simulink model "Myp6LinearIntegralObserverFeed"  (R2021b)
settings: Solver=ode4  StartTime=0.0  StopTime=TIME_SIM  FixedStep=STEP_SIZE  RelTol=1e-3
values from neighbouring files (symbols this model uses):
  Aa = [-0.329723564087  0.00108308678514  -14.6666835708; 119.959269051  -1.23669349537  16746.7578957; 1  -0.0103092783505  0]    [LinearModel.mat]
  Bb = [-1.10657474768  0; 0  -0.0018722524695; 0  0]    [LinearModel.mat]
  Bv = [0.0209040137669 0 0]    [LinearModel.mat]
  Dd = [0  0; 0  0.0001229087]    [LinearModel.mat]
  xOP = [1.2671 122.9087 0.00454800621385]    [LinearModel.mat]
undefined symbols (not defined in the file or in its folder): Cc0, Ff, Gg, K_FSF, Ki, L, Ts
settings Model: Creator=tanzc  LastModifiedBy=tanzc
settings DataIOCC: SaveFormat=Array  ReturnWorkspaceOutputs=off

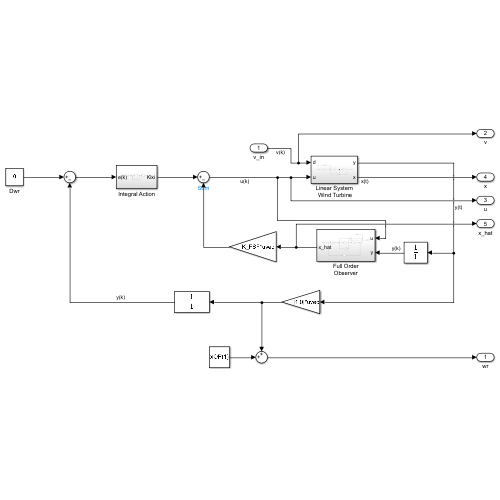
[thumbnail: Simulink's stored preview of the top-level diagram]
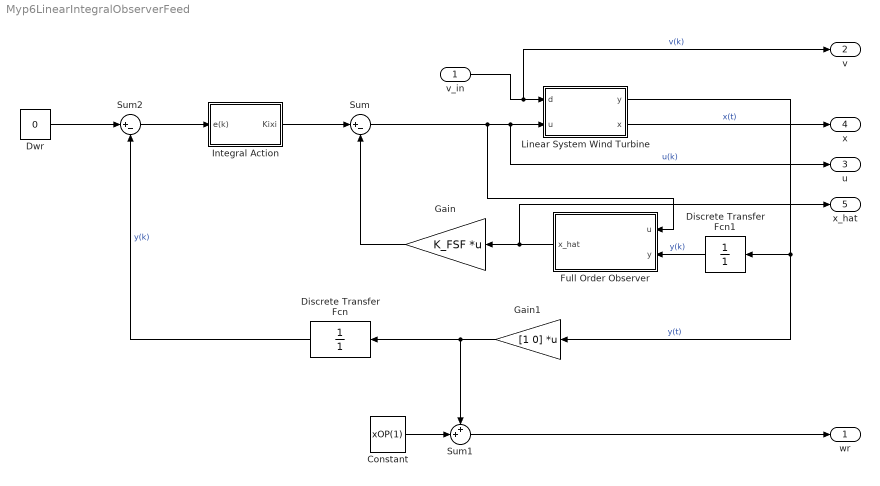
== system Myp6LinearIntegralObserverFeed ==
  v_in : Inport
  Constant : Constant  Value=xOP(1)
  Discrete Transfer Fcn : DiscreteTransferFcn  Denominator=1  SampleTime=Ts
  Discrete Transfer Fcn1 : DiscreteTransferFcn  Denominator=1  SampleTime=Ts
  Dwr : Constant  Value=0  SampleTime=Ts
  Full Order Observer : Subsystem
  Gain : Gain  Gain=K_FSF  Multiplication=Matrix(K*u) (u vector)
  Gain1 : Gain  Gain=[1 0]  Multiplication=Matrix(K*u) (u vector)
  Integral Action : Subsystem
  Linear System Wind Turbine : Subsystem
  Sum : Sum  Inputs=|+-
  Sum1 : Sum  Inputs=++|
  Sum2 : Sum  Inputs=|+-
  wr : Outport
  v : Outport  Port=2
  u : Outport  Port=3
  x : Outport  Port=4
  x_hat : Outport  Port=5
  wires:
  Gain/1 -> Sum/2
  Sum/1 -> Full Order Observer/1(u), Linear System Wind Turbine/2(u), u/1  "u(k)"
  v_in/1 -> v/1, Linear System Wind Turbine/1(d)  "v(k)"
  Dwr/1 -> Sum2/1
  Discrete Transfer Fcn/1 -> Sum2/2  "y(k)"
  Linear System Wind Turbine/1(y) -> Discrete Transfer Fcn1/1, Gain1/1  "y(t)"
  Sum2/1 -> Integral Action/1(e(k))
  Integral Action/1(Kixi) -> Sum/1
  Discrete Transfer Fcn1/1 -> Full Order Observer/2(y)  "y(k)"
  Full Order Observer/1(x_hat) -> x_hat/1, Gain/1
  Gain1/1 -> Sum1/1, Discrete Transfer Fcn/1
  Constant/1 -> Sum1/2
  Sum1/1 -> wr/1
  Linear System Wind Turbine/2(x) -> x/1  "x(t)"

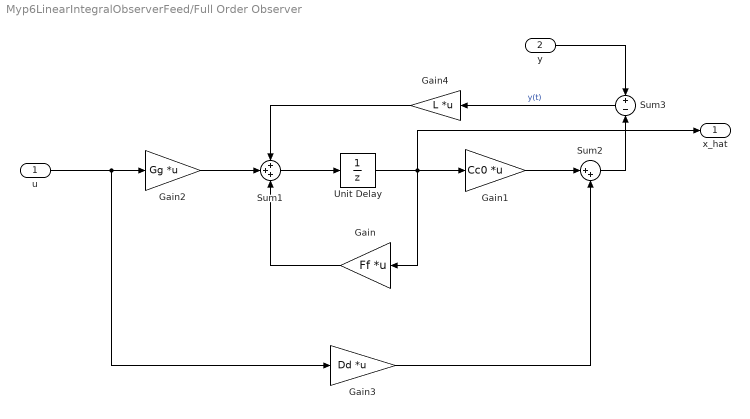
== system Myp6LinearIntegralObserverFeed/Full Order Observer ==
  u : Inport
  y : Inport  Port=2
  Gain : Gain  Gain=Ff  Multiplication=Matrix(K*u) (u vector)
  Gain1 : Gain  Gain=Cc0  Multiplication=Matrix(K*u) (u vector)
  Gain2 : Gain  Gain=Gg  Multiplication=Matrix(K*u) (u vector)
  Gain3 : Gain  Gain=Dd  Multiplication=Matrix(K*u) (u vector)
  Gain4 : Gain  Gain=L  Multiplication=Matrix(K*u) (u vector)
  Sum1 : Sum  Inputs=+++
  Sum2 : Sum  Inputs=|++
  Sum3 : Sum  Inputs=+-
  Unit Delay : UnitDelay  SampleTime=Ts  HasFrameUpgradeWarning=on
  x_hat : Outport
  wires:
  y/1 -> Sum3/1
  Gain1/1 -> Sum2/1
  Unit Delay/1 -> x_hat/1, Gain/1, Gain1/1
  Gain2/1 -> Sum1/2
  Sum2/1 -> Sum3/2
  u/1 -> Gain3/1, Gain2/1
  Gain3/1 -> Sum2/2
  Gain/1 -> Sum1/3
  Gain4/1 -> Sum1/1
  Sum1/1 -> Unit Delay/1
  Sum3/1 -> Gain4/1  "y(t)"

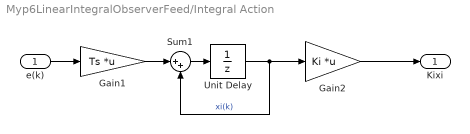
== system Myp6LinearIntegralObserverFeed/Integral Action ==
  e(k) : Inport
  Gain1 : Gain  Gain=Ts  Multiplication=Matrix(K*u) (u vector)
  Gain2 : Gain  Gain=Ki  Multiplication=Matrix(K*u) (u vector)
  Sum1 : Sum  Inputs=|++
  Unit Delay : UnitDelay  SampleTime=Ts  HasFrameUpgradeWarning=on
  Kixi : Outport
  wires:
  e(k)/1 -> Gain1/1
  Unit Delay/1 -> Sum1/2, Gain2/1  "xi(k)"
  Gain1/1 -> Sum1/1
  Gain2/1 -> Kixi/1
  Sum1/1 -> Unit Delay/1

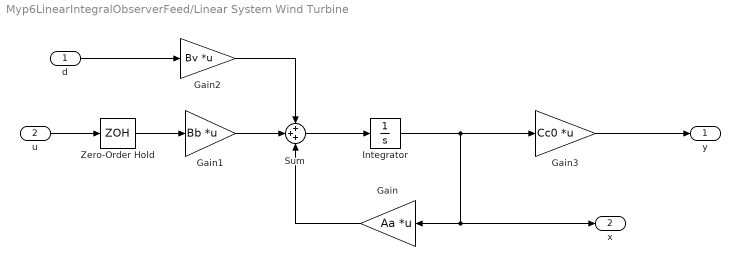
== system Myp6LinearIntegralObserverFeed/Linear System Wind Turbine ==
  d : Inport
  u : Inport  Port=2
  Gain : Gain  Gain=Aa  Multiplication=Matrix(K*u) (u vector)
  Gain1 : Gain  Gain=Bb  Multiplication=Matrix(K*u) (u vector)
  Gain2 : Gain  Gain=Bv  Multiplication=Matrix(K*u) (u vector)
  Gain3 : Gain  Gain=Cc0  Multiplication=Matrix(K*u) (u vector)
  Integrator : Integrator
  Sum : Sum  Inputs=+++
  Zero-Order Hold : ZeroOrderHold  SampleTime=-1
  y : Outport
  x : Outport  Port=2
  wires:
  Gain3/1 -> y/1
  d/1 -> Gain2/1
  Integrator/1 -> Gain3/1, x/1, Gain/1
  Gain2/1 -> Sum/1
  Gain/1 -> Sum/3
  Gain1/1 -> Sum/2
  Sum/1 -> Integrator/1
  Zero-Order Hold/1 -> Gain1/1
  u/1 -> Zero-Order Hold/1
